simulink model "PubIfDecisionTOS_MDL"  (R2020b)
settings: configuration reference "DspaceConfig" (kept outside this file)
PostLoadFcn:
  | if any(exist('dsrtsu_mdlpostloadfcn', 'file') ~= 0), dsrtsu_mdlpostloadfcn('Execute', bdroot); end
InitFcn:
  | , if any(exist('dsmpb_private', 'file') ~= 0), dsmpb_private('dsmpb_mdlclblib', 'Init', bdroot); end,
undefined symbols (not defined in the file or in its folder): C_TOS_ACCEgoRAxletoFbumplength_m, C_TOS_ACCTargetFront_Flag, C_TOS_AEBJAPedObjDxThre_Val, C_TOS_AEBJAPedObjDyThre_Val, C_TOS_AEBJATargetSize_Val, C_TOS_AEBJAVehObjDxThre_Val, C_TOS_AEBJAVehObjDyThre_Val, C_TOS_AEBJuncPedTargetSize_Val, C_TOS_AEBLatObjDxThre_Val, C_TOS_AEBLatPedDyThre_Val, C_TOS_AEBLatTargetSize_Val, C_TOS_AEBLongTargetInEgoFront_Flag, C_TOS_axAbsGround_Parameter, C_TOS_CameraConfirmedFlag, C_TOS_CNsubjWidth, C_TOS_CurrentLaneCoreMinWidth_Val, C_TOS_CutInProb_Val_Zero, C_TOS_CutOutProb_Val_Zero, C_TOS_D2R_Val, C_TOS_DefaultValueObjectToCenterLine_dy, C_TOS_EgoCarWidth_Val, C_TOS_EgoDxRefPoint_m, C_TOS_EgoRAxletoFbumplength_m, C_TOS_HalfWidthVehicle_Con, C_TOS_HWA_CurrentLaneFlag, C_TOS_HWA_LeftLaneFlag, C_TOS_HWA_MovingDir_Vaild, C_TOS_HWA_MovState_Vaild, C_TOS_HWA_RightLaneFlag, C_TOS_LaneLineCourseErrorFront, C_TOS_LaneLineCourseErrorRear, C_TOS_MotorbikeDefaultWidth_m, C_TOS_NumberOfEffectiveTargets, C_TOS_Obj_Age_Val, C_TOS_Objdx_Constraint_Val, C_TOS_ObjectDefaultWidth_m, C_TOS_ObjInCurrentLane_Val, C_TOS_ObjInCurrentLaneValid, C_TOS_ObjInLeftLaneValid, C_TOS_ObjInRightLaneValid, C_TOS_ObjNotInCurrentLane_Val, C_TOS_ObjNotREElementType, C_TOS_ObjPredictDis_dy_ConstantVal_Zeros, C_TOS_ObjToCenterLine_ConstantVal_Zeros, C_TOS_OFMObjIDInvilad_Val, C_TOS_PIL_LatDisCons_Val_zero, C_TOS_PIL_ObjectCutInFlag_b, C_TOS_PIL_ObjectCutOutFlag_b, C_TOS_PIL_ObjLaneProb_al_Val, C_TOS_PP_ObjFusType_FC_Confirm_b, C_TOS_PP_ObjFusType_FC_FR_Confirm_b, C_TOS_PP_ObjFusType_FR_Confirm_b, C_TOS_RE_80BoolDefault_Val, C_TOS_RE_80Single181Default_Val, C_TOS_RE_80Single255Default_Val, C_TOS_RE_80Uint8Default_Val, C_TOS_RE_D2R, C_TOS_RE_D_180_Val, C_TOS_RE_InvalidObjectID_Val, C_TOS_RE_InvalidTargetChainDir_Val ... (+142)
libraries: simulink x1650, TOS_LIB x361, canfdmsglib x14
(part 17 of 69)

== system PubIfDecisionTOS_MDL/TOS_20201112/TOS_2012080320/PP1128/AAT-AdditionalAttributes/PP_ObjectToCenterLine_dy/PP_ObjectToCenterLine_vyc/PP_ObjectToCenterLine_vyc_Filt ==
  TOS_OFMObjValid_Flag : Inport
  Object_ID : Inport  Port=2  OutDataTypeStr=uint8
  Object_Age : Inport  Port=3
  PP_ObjectToCenterLine_vyc : Inport  Port=4
  ObjectToCenterLine_vyc : Subsystem
  Unit Delay : UnitDelay  InitialCondition=zeros(80,1)  SampleTime=-1  HasFrameUpgradeWarning=on
      settings: AttributesFormatString=initVal = zeros(80,1)
  Unit Delay1 : UnitDelay  InitialCondition=ones(80,1)*255  SampleTime=-1  HasFrameUpgradeWarning=on
      settings: AttributesFormatString=initVal = ones(80,1)*255
  PP_ObjectToCenterLine_vyc_Filt : Outport  OutDataTypeStr=single
  wires:
  TOS_OFMObjValid_Flag/1 -> ObjectToCenterLine_vyc/4(TOS_OFMObjValid_Flag)
  Object_Age/1 -> ObjectToCenterLine_vyc/6(Object_Age)
  PP_ObjectToCenterLine_vyc/1 -> ObjectToCenterLine_vyc/3(PP_ObjectToCenterLine_vyc)
  ObjectToCenterLine_vyc/2(PP_ObjectToCenterLine_vyc_Filt) -> PP_ObjectToCenterLine_vyc_Filt/1, Unit Delay1/1
  Unit Delay1/1 -> ObjectToCenterLine_vyc/2(PP_ObjectToCenterLine_vyc_Filt_K1)
  Object_ID/1 -> ObjectToCenterLine_vyc/5(Object_ID)
  ObjectToCenterLine_vyc/1(Obj_ID) -> Unit Delay/1
  Unit Delay/1 -> ObjectToCenterLine_vyc/1(ObjectID_Filt_K1)

== system PubIfDecisionTOS_MDL/TOS_20201112/TOS_2012080320/PP1128/AAT-AdditionalAttributes/PP_SignalProcessing/PP_SignalProcessing/CamareConfirmSignalProcessing ==
  note: PP_CamareConfirmSignalProcessing
      |
      | 是否摄像头确认信号（AEB）
      |
      | fun1:有摄像头、前雷达参与
  Object_FusType : Inport
  Data Type Conversion : DataTypeConversion  OutDataTypeStr=Enum: OFM_OBJ_FUSTYPE
  Enumerated Constant : simulink/Sources/Enumerated Constant  OutDataTypeStr=Enum: OFM_OBJ_FUSTYPE  Value=OFM_OBJ_FUSTYPE.FC_FR  SampleTime=inf
      settings: AttributesFormatString=OFM_OBJ_FUSTYPE.FC_FR = 3
  Enumerated Constant1 : simulink/Sources/Enumerated Constant  OutDataTypeStr=Enum: OFM_OBJ_FUSTYPE  Value=OFM_OBJ_FUSTYPE.FC_FR_CL  SampleTime=inf
      settings: AttributesFormatString=OFM_OBJ_FUSTYPE.FC_FR_CL=7
  Enumerated Constant10 : simulink/Sources/Enumerated Constant  OutDataTypeStr=Enum: OFM_OBJ_FUSTYPE  Value=OFM_OBJ_FUSTYPE.FC_FR_CR_BR  SampleTime=inf
      settings: AttributesFormatString=OFM_OBJ_FUSTYPE.FC_FR_CR_BR=43
  Enumerated Constant11 : simulink/Sources/Enumerated Constant  OutDataTypeStr=Enum: OFM_OBJ_FUSTYPE  Value=OFM_OBJ_FUSTYPE.FC_FR_CL_CR_BR  SampleTime=inf
      settings: AttributesFormatString=OFM_OBJ_FUSTYPE.FC_FR_CL_CR_BR=47
  Enumerated Constant12 : simulink/Sources/Enumerated Constant  OutDataTypeStr=Enum: OFM_OBJ_FUSTYPE  Value=OFM_OBJ_FUSTYPE.FC_FR_BL_BR  SampleTime=inf
      settings: AttributesFormatString=OFM_OBJ_FUSTYPE.FC_FR_BL_BR=51
  Enumerated Constant13 : simulink/Sources/Enumerated Constant  OutDataTypeStr=Enum: OFM_OBJ_FUSTYPE  Value=OFM_OBJ_FUSTYPE.FC_FR_CR_BL_BR  SampleTime=inf
      settings: AttributesFormatString=OFM_OBJ_FUSTYPE.FC_FR_CR_BL_BR=59
  Enumerated Constant14 : simulink/Sources/Enumerated Constant  OutDataTypeStr=Enum: OFM_OBJ_FUSTYPE  Value=OFM_OBJ_FUSTYPE.FC_FR_CL_BL_BR  SampleTime=inf
      settings: AttributesFormatString=OFM_OBJ_FUSTYPE.FC_FR_CL_BL_BR=55
  Enumerated Constant15 : simulink/Sources/Enumerated Constant  OutDataTypeStr=Enum: OFM_OBJ_FUSTYPE  Value=OFM_OBJ_FUSTYPE.FC_FR_CL_CR_BL_BR  SampleTime=inf
      settings: AttributesFormatString=OFM_OBJ_FUSTYPE.FC_FR_CL_CR_BL_BR=63
  Enumerated Constant2 : simulink/Sources/Enumerated Constant  OutDataTypeStr=Enum: OFM_OBJ_FUSTYPE  Value=OFM_OBJ_FUSTYPE.FC_FR_CR  SampleTime=inf
      settings: AttributesFormatString=OFM_OBJ_FUSTYPE.FC_FR_CR=11
  Enumerated Constant3 : simulink/Sources/Enumerated Constant  OutDataTypeStr=Enum: OFM_OBJ_FUSTYPE  Value=OFM_OBJ_FUSTYPE.FC_FR_CL_CR  SampleTime=inf
      settings: AttributesFormatString=OFM_OBJ_FUSTYPE.FC_FR_CL_CR=15
  Enumerated Constant4 : simulink/Sources/Enumerated Constant  OutDataTypeStr=Enum: OFM_OBJ_FUSTYPE  Value=OFM_OBJ_FUSTYPE.FC_FR_BL  SampleTime=inf
      settings: AttributesFormatString=OFM_OBJ_FUSTYPE.FC_FR_BL=19
  Enumerated Constant5 : simulink/Sources/Enumerated Constant  OutDataTypeStr=Enum: OFM_OBJ_FUSTYPE  Value=OFM_OBJ_FUSTYPE.FC_FR_CL_BL  SampleTime=inf
      settings: AttributesFormatString=OFM_OBJ_FUSTYPE.FC_FR_CL_BL=23
  Enumerated Constant6 : simulink/Sources/Enumerated Constant  OutDataTypeStr=Enum: OFM_OBJ_FUSTYPE  Value=OFM_OBJ_FUSTYPE.FC_FR_CR_BL  SampleTime=inf
      settings: AttributesFormatString=OFM_OBJ_FUSTYPE.FC_FR_CR_BL=27
  Enumerated Constant7 : simulink/Sources/Enumerated Constant  OutDataTypeStr=Enum: OFM_OBJ_FUSTYPE  Value=OFM_OBJ_FUSTYPE.FC_FR_CL_CR_BL  SampleTime=inf
      settings: AttributesFormatString=OFM_OBJ_FUSTYPE.FC_FR_CL_CR_BL=31
  Enumerated Constant8 : simulink/Sources/Enumerated Constant  OutDataTypeStr=Enum: OFM_OBJ_FUSTYPE  Value=OFM_OBJ_FUSTYPE.FC_FR_BR  SampleTime=inf
      settings: AttributesFormatString=OFM_OBJ_FUSTYPE.FC_FR_BR=35
  Enumerated Constant9 : simulink/Sources/Enumerated Constant  OutDataTypeStr=Enum: OFM_OBJ_FUSTYPE  Value=OFM_OBJ_FUSTYPE.FC_FR_CL_BR  SampleTime=inf
      settings: AttributesFormatString=OFM_OBJ_FUSTYPE.FC_FR_CL_BR=39
  Logical Operator{1..15} (15 alike) : Logic  Operator=OR  AllPortsSameDT=off  OutDataTypeStr=boolean
  Relational Operator{1..16} (16 alike) : RelationalOperator  Operator===  OutDataTypeStr=boolean  RndMeth=Nearest
  PP_CamareConfirmSignalProcessing : Outport
  wires:
  Enumerated Constant1/1 -> Relational Operator12/2
  Relational Operator12/1 -> Logical Operator8/2
  Enumerated Constant2/1 -> Relational Operator13/2
  Enumerated Constant3/1 -> Relational Operator15/2
  Relational Operator15/1 -> Logical Operator9/2
  Relational Operator14/1 -> Logical Operator8/1
  Logical Operator15/1 -> PP_CamareConfirmSignalProcessing/1
  Relational Operator13/1 -> Logical Operator9/1
  Logical Operator8/1 -> Logical Operator10/1
  Logical Operator9/1 -> Logical Operator10/2
  Enumerated Constant/1 -> Relational Operator14/2
  Object_FusType/1 -> Data Type Conversion/1
  Enumerated Constant4/1 -> Relational Operator3/2
  Enumerated Constant7/1 -> Relational Operator4/2
  Enumerated Constant6/1 -> Relational Operator2/2
  Enumerated Constant5/1 -> Relational Operator1/2
  Enumerated Constant9/1 -> Relational Operator5/2
  Enumerated Constant10/1 -> Relational Operator6/2
  Enumerated Constant11/1 -> Relational Operator8/2
  Enumerated Constant8/1 -> Relational Operator7/2
  Enumerated Constant12/1 -> Relational Operator11/2
  Enumerated Constant15/1 -> Relational Operator16/2
  Data Type Conversion/1 -> Relational Operator14/1, Relational Operator12/1, Relational Operator3/1, Relational Operator1/1, Relational Operator2/1, Relational Operator4/1, Relational Operator7/1, Relational Operator5/1, Relational Operator6/1, Relational Operator8/1, Relational Operator11/1, Relational Operator9/1, Relational Operator10/1, Relational Operator16/1, Relational Operator15/1, Relational Operator13/1
  Enumerated Constant13/1 -> Relational Operator10/2
  Enumerated Constant14/1 -> Relational Operator9/2
  Relational Operator3/1 -> Logical Operator1/1
  Relational Operator1/1 -> Logical Operator1/2
  Relational Operator2/1 -> Logical Operator2/1
  Relational Operator4/1 -> Logical Operator2/2
  Relational Operator9/1 -> Logical Operator4/2
  Relational Operator11/1 -> Logical Operator4/1
  Relational Operator8/1 -> Logical Operator3/2
  Relational Operator6/1 -> Logical Operator3/1
  Relational Operator7/1 -> Logical Operator5/1
  Relational Operator5/1 -> Logical Operator5/2
  Relational Operator10/1 -> Logical Operator6/1
  Relational Operator16/1 -> Logical Operator6/2
  Logical Operator2/1 -> Logical Operator12/2
  Logical Operator1/1 -> Logical Operator12/1
  Logical Operator5/1 -> Logical Operator13/1
  Logical Operator3/1 -> Logical Operator13/2
  Logical Operator6/1 -> Logical Operator7/2
  Logical Operator4/1 -> Logical Operator7/1
  Logical Operator10/1 -> Logical Operator11/1
  Logical Operator12/1 -> Logical Operator11/2
  Logical Operator13/1 -> Logical Operator14/1
  Logical Operator7/1 -> Logical Operator14/2
  Logical Operator11/1 -> Logical Operator15/1
  Logical Operator14/1 -> Logical Operator15/2

== system PubIfDecisionTOS_MDL/TOS_20201112/TOS_2012080320/PP1128/AAT-AdditionalAttributes/PP_SignalProcessing/PP_SignalProcessing/MovingState_SignalProcessing ==
  Object_MovingState : Inport
  MovingState_SignalProcessing_V2011120315 : Subsystem
  MovingState_SignalProcessing_V2011130316 : Subsystem
  PP_MovingStateSignalProcessing : Outport
  PP_MovingState_AEB_SignalProcessing : Outport  Port=2
  wires:
  MovingState_SignalProcessing_V2011130316/1(PP_MovingStateSignalProcessing) -> PP_MovingStateSignalProcessing/1
  Object_MovingState/1 -> MovingState_SignalProcessing_V2011120315/1(Object_MovingState), MovingState_SignalProcessing_V2011130316/1(Object_MovingState)
  MovingState_SignalProcessing_V2011120315/1(PP_MovingStateSignalProcessing) -> PP_MovingState_AEB_SignalProcessing/1

== system PubIfDecisionTOS_MDL/TOS_20201112/TOS_2012080320/PP1128/AAT-AdditionalAttributes/PP_SignalProcessing/PP_SignalProcessing/ObjFusTypeConfirm ==
  Object_FusType : Inport
  Data Type Conversion : DataTypeConversion  OutDataTypeStr=Enum: OFM_OBJ_FUSTYPE
  FC_FR_other : Subsystem
  FC_other : Subsystem
  FR_other : Subsystem
  ObjFusType : Subsystem  Commented=on
  ObjFusType_FC_FR_Confirm : Outport
  ObjFusType_FR_Confirm : Outport  Port=2
  ObjFusType_FC_Confirm : Outport  Port=3
  wires:
  Object_FusType/1 -> Data Type Conversion/1
  Data Type Conversion/1 -> FC_other/1(Object_FusType), FR_other/1(Object_FusType), FC_FR_other/1(Object_FusType)
  FC_FR_other/1(FC_FR_other) -> ObjFusType_FC_FR_Confirm/1
  FR_other/1(FR_Other) -> ObjFusType_FR_Confirm/1
  FC_other/1(FC_other) -> ObjFusType_FC_Confirm/1

== system PubIfDecisionTOS_MDL/TOS_20201112/TOS_2012080320/PP1128/AAT-AdditionalAttributes/PP_SignalProcessing/PP_SignalProcessing/ObjMovingDirSignalProcessing ==
  Object_MovingOrientation : Inport
  Compare To Constant : simulink/Logic and Bit Operations/Compare To Constant  relop===  const=OFM_OBJ_ORIENTATION_E.NORTH  OutDataTypeStr=boolean
      settings: AttributesFormatString=OFM_OBJ_ORIENTATION_E.NORTH = 9
  Compare To Constant3 : simulink/Logic and Bit Operations/Compare To Constant  relop===  const=OFM_OBJ_ORIENTATION_E.SOUTH  OutDataTypeStr=boolean
      settings: AttributesFormatString=OFM_OBJ_ORIENTATION_E.SOUTH = 5
  Compare To Constant4 : simulink/Logic and Bit Operations/Compare To Constant  relop===  const=OFM_OBJ_ORIENTATION_E.WEST  OutDataTypeStr=boolean
      settings: AttributesFormatString=OFM_OBJ_ORIENTATION_E.WEST = 7
  Compare To Constant5 : simulink/Logic and Bit Operations/Compare To Constant  relop===  const=OFM_OBJ_ORIENTATION_E.EAST  OutDataTypeStr=boolean
      settings: AttributesFormatString=OFM_OBJ_ORIENTATION_E.EAST = 3
  Data Type Conversion1 : DataTypeConversion  OutDataTypeStr=uint8
  Data Type Conversion2 : DataTypeConversion  OutDataTypeStr=Enum: OFM_OBJ_ORIENTATION_E
  Enumerated Constant : simulink/Sources/Enumerated Constant  OutDataTypeStr=Enum: ObjectMovingOrientation_E  Value=ObjectMovingOrientation_E.SameDir  SampleTime=inf
      settings: AttributesFormatString=ObjectMovingOrientation_E.SameDir = 1
  Enumerated Constant1 : simulink/Sources/Enumerated Constant  OutDataTypeStr=Enum: ObjectMovingOrientation_E  Value=ObjectMovingOrientation_E.OnComingDir  SampleTime=inf
      settings: AttributesFormatString=ObjectMovingOrientation_E.OnComingDir = 2
  Enumerated Constant2 : simulink/Sources/Enumerated Constant  OutDataTypeStr=Enum: ObjectMovingOrientation_E  Value=ObjectMovingOrientation_E.Crossing  SampleTime=inf
      settings: AttributesFormatString=ObjectMovingOrientation_E.Crossing = 3
  Enumerated Constant3 : simulink/Sources/Enumerated Constant  OutDataTypeStr=Enum: ObjectMovingOrientation_E  Value=ObjectMovingOrientation_E.UnknownDir  SampleTime=inf
      settings: AttributesFormatString=ObjectMovingOrientation_E.UnknownDir = 0
  Logical Operator6 : Logic  Operator=OR  AllPortsSameDT=off  OutDataTypeStr=boolean
  Switch : Switch  Criteria=u2 ~= 0
  Switch1 : Switch  Criteria=u2 ~= 0
  Switch2 : Switch  Criteria=u2 ~= 0
  PP_ObjMovingDirSignalProcessing : Outport
  wires:
  Switch/1 -> Data Type Conversion1/1
  Enumerated Constant3/1 -> Switch2/3
  Switch1/1 -> Switch/3
  Switch2/1 -> Switch1/3
  Enumerated Constant2/1 -> Switch2/1
  Enumerated Constant1/1 -> Switch1/1
  Logical Operator6/1 -> Switch2/2
  Compare To Constant3/1 -> Switch1/2
  Compare To Constant4/1 -> Logical Operator6/1
  Data Type Conversion2/1 -> Compare To Constant/1, Compare To Constant3/1, Compare To Constant5/1, Compare To Constant4/1
  Compare To Constant5/1 -> Logical Operator6/2
  Enumerated Constant/1 -> Switch/1
  Compare To Constant/1 -> Switch/2
  Object_MovingOrientation/1 -> Data Type Conversion2/1
  Data Type Conversion1/1 -> PP_ObjMovingDirSignalProcessing/1

== system PubIfDecisionTOS_MDL/TOS_20201112/TOS_2012080320/PP1128/AAT-AdditionalAttributes/PP_SignalProcessing/PP_SignalProcessing/ObjToEgoCarFrontbump ==
  note: 目标到自车前保之间距离
  Object_Dx : Inport
  Constant1 : Constant  Value=C_TOS_ACCEgoRAxletoFbumplength_m  OutDataTypeStr=single
      settings: AttributesFormatString=C_TOS_ACCEgoRAxletoFbumplength_m = 3.93 m
  Subtract : Sum  Inputs=+-
  PP_ObjToEgoCarFrontbump : Outport
  wires:
  Object_Dx/1 -> Subtract/1
  Subtract/1 -> PP_ObjToEgoCarFrontbump/1
  Constant1/1 -> Subtract/2

== system PubIfDecisionTOS_MDL/TOS_20201112/TOS_2012080320/PP1128/AAT-AdditionalAttributes/PP_SignalProcessing/PP_SignalProcessing/axAbsGround ==
  note: Fun：计算目标相对于大地的绝对加速度(ACC)
      |
      | fun1:目标绝对加速度 = 目标相对加速度（融合输出）+ 自车加速度
      | fun2: 当目标状态为STATIONARY、STOPPED时，输出目标绝对加速度为0
      |
      |
      | （目标相对加速度 = 目标加速度 - 自车加速度）
  Object_AX : Inport
  axvRefMs2 : Inport  Port=2
  Object_MovingState : Inport  Port=3
  Add : Sum
  Compare To Constant : simulink/Logic and Bit Operations/Compare To Constant  relop===  const=OFM_OBJ_MOVINGSTATE_E.STATIONARY  OutDataTypeStr=boolean
      settings: AttributesFormatString=OFM_OBJ_MOVINGSTATE_E.STATIONARY = 3
  Compare To Constant1 : simulink/Logic and Bit Operations/Compare To Constant  relop===  const=OFM_OBJ_MOVINGSTATE_E.STOPPED  OutDataTypeStr=boolean
      settings: AttributesFormatString=OFM_OBJ_MOVINGSTATE_E.STOPPED = 4
  Constant1 : Constant  Value=C_TOS_axAbsGround_Parameter  OutDataTypeStr=single
      settings: AttributesFormatString=C_TOS_axAbsGround_Parameter = 0
  Data Type Conversion : DataTypeConversion  OutDataTypeStr=Enum: OFM_OBJ_MOVINGSTATE_E
  Logical Operator : Logic  Operator=OR  AllPortsSameDT=off  OutDataTypeStr=boolean
  Switch1 : Switch  Criteria=u2 ~= 0
  PP_axAbsGround : Outport
  wires:
  Compare To Constant1/1 -> Logical Operator/2
  axvRefMs2/1 -> Add/2
  Data Type Conversion/1 -> Compare To Constant1/1, Compare To Constant/1
  Object_AX/1 -> Add/1
  Compare To Constant/1 -> Logical Operator/1
  Object_MovingState/1 -> Data Type Conversion/1
  Switch1/1 -> PP_axAbsGround/1
  Constant1/1 -> Switch1/1
  Add/1 -> Switch1/3
  Logical Operator/1 -> Switch1/2

== system PubIfDecisionTOS_MDL/TOS_20201112/TOS_2012080320/PP1128/AAT-AdditionalAttributes/RoadEdge/RE_2020_12_07/RoadEdge_V2 ==
  OFM_Signal : Inport  BusOutputAsStruct=on
  vxvRefMs : Inport  Port=2  OutDataTypeStr=single  PortDimensions=1  BusOutputAsStruct=on
  Bus Selector : BusSelector  OutputSignals=RE_EgoLeftTargetChainStartIndex
  Bus Selector1 : BusSelector  OutputSignals=RE_EgoRightTargetChainStartIndex
  Bus Selector2 : BusSelector  OutputSignals=RE_EgoLeftEdgeGroupChainStartIndex
  Bus Selector3 : BusSelector  OutputSignals=RE_EgoRightEdgeGroupChainStartIndex
  Bus Selector4 : BusSelector  OutputSignals=RE_EgoRightStationaryObjectsSortIndex
  Bus Selector5 : BusSelector  OutputSignals=RE_EgoLeftStationaryObjectsSortIndex
  RoadEdgeElementFinalJudge : Subsystem
  RoadEdgeElementType : Subsystem
  RoadEdgeGroupChain : Subsystem
  SelectStationaryObjects : Subsystem
  TargetChain : Subsystem
  Unit Delay1 : UnitDelay  SampleTime=-1  HasFrameUpgradeWarning=on
  Unit Delay2 : UnitDelay  SampleTime=-1  HasFrameUpgradeWarning=on
  RE_EdgeElementType : Outport
  RE_StationaryObjectFlag : Outport  Port=2
  RE_EgoLeftTargetChainStartIndex : Outport  Port=3
  RE_EgoRightTargetChainStartIndex : Outport  Port=4
  RE_EgoLeftEdgeGroupChainStartIndex : Outport  Port=5
  RE_EgoRightEdgeGroupChainStartIndex : Outport  Port=6
  RE_EgoLeftStationaryObjectsSortIndex : Outport  Port=7
  RE_EgoRightStationaryObjectsSortIndex : Outport  Port=8
  RE_EdgeElementID : Outport  Port=9
  wires:
  vxvRefMs/1 -> RoadEdgeGroupChain/6(vxvRefMs), RoadEdgeElementFinalJudge/5(vxvRefMs)
  SelectStationaryObjects/1(RE_StationaryObjectsSortIndex) -> Bus Selector5/1, Bus Selector4/1, TargetChain/1(RE_StillObjectsSortIndex)  "RE_StationaryObjectsSortIndex"
  TargetChain/1(RE_StillObjectSortIndex) -> RoadEdgeGroupChain/1(RE_StillObjectSortIndex)  "RE_StillObjectSortIndex"
  TargetChain/2(RE_EgoLeftTargetChainInfor) -> RoadEdgeGroupChain/2(RE_EgoLeftTargetChainInfor), Bus Selector/1  "RE_EgoLeftTargetChainInfor"
  TargetChain/3(RE_EgoRightTargetChainInfor) -> RoadEdgeGroupChain/3(RE_EgoRightTargetChainInfor), Bus Selector1/1  "RE_EgoRightTargetChainInfor"
  TargetChain/4(RE_TargetTheta) -> RoadEdgeGroupChain/4(RE_TargetTheta)  "RE_TargetTheta"
  RoadEdgeGroupChain/1(RE_EgoLeftEdgeGroupChainInfor) -> Bus Selector2/1, RoadEdgeElementFinalJudge/1(RE_EgoLeftEdgeGroupChainInfor)  "RE_EgoLeftEdgeGroupChainInfor"
  RoadEdgeElementType/1(RE_EdgeElementType) -> RE_EdgeElementType/1  "RE_EdgeElementType"
  RoadEdgeGroupChain/2(RE_EgoRightEdgeGroupChainInfor) -> Bus Selector3/1, RoadEdgeElementFinalJudge/2(RE_EgoRightEdgeGroupChainInfor)  "RE_EgoRightEdgeGroupChainInfor"
  RoadEdgeGroupChain/3(RE_Target_Theta) -> RoadEdgeElementFinalJudge/3(RE_Target_Theta)  "RE_Target_Theta"
  RoadEdgeGroupChain/4(REStillObjectSortIndex) -> RoadEdgeElementFinalJudge/4(REStillObjectSortIndex)  "REStillObjectSortIndex"
  RoadEdgeElementFinalJudge/1(RE_EgoLeft_EdgeElementType) -> RoadEdgeElementType/1(RE_EgoLeft_EdgeElementType)  "RE_EgoLeft_EdgeElementType"
  RoadEdgeElementFinalJudge/2(RE_EgoRight_EdgeElementType) -> RoadEdgeElementType/2(RE_EgoRight_EdgeElementType)  "RE_EgoRight_EdgeElementType"
  SelectStationaryObjects/2(RE_StationaryObjectFlag) -> RE_StationaryObjectFlag/1
  Bus Selector/1 -> RE_EgoLeftTargetChainStartIndex/1  "<RE_EgoLeftTargetChainStartIndex>"
  Bus Selector1/1 -> RE_EgoRightTargetChainStartIndex/1  "<RE_EgoRightTargetChainStartIndex>"
  Bus Selector3/1 -> RE_EgoRightEdgeGroupChainStartIndex/1  "<RE_EgoRightEdgeGroupChainStartIndex>"
  Bus Selector2/1 -> RE_EgoLeftEdgeGroupChainStartIndex/1  "<RE_EgoLeftEdgeGroupChainStartIndex>"
  Bus Selector4/1 -> RE_EgoRightStationaryObjectsSortIndex/1  "<RE_EgoRightStationaryObjectsSortIndex>"
  Bus Selector5/1 -> RE_EgoLeftStationaryObjectsSortIndex/1  "<RE_EgoLeftStationaryObjectsSortIndex>"
  RoadEdgeElementType/2(RE_EdgeElementID) -> [RE_EdgeElementID], RE_EdgeElementID/1  "RE_EdgeElementID"
  RoadEdgeElementFinalJudge/3(RE_EgoLeft_EdgeElementID) -> RoadEdgeElementType/3(RE_EgoLeft_EdgeElementID)  "RE_EgoLeft_EdgeElementID"
  RoadEdgeElementFinalJudge/4(RE_EgoRight_EdgeElementID) -> RoadEdgeElementType/4(RE_EgoRight_EdgeElementID)  "RE_EgoRight_EdgeElementID"
  OFM_Signal/1 -> RoadEdgeGroupChain/5(OFM_Signal), RoadEdgeElementType/5(OFM_Signal), RoadEdgeElementFinalJudge/7(OFM_Signal), TargetChain/2(OFM_Signal), SelectStationaryObjects/1(OFM_Signal)
  [RE_EdgeElementID] -> Unit Delay2/1
  [RE_EdgeElementID] -> Unit Delay1/1
  Unit Delay2/1 -> TargetChain/3(RE_EdgeElementID_K1)
  Unit Delay1/1 -> RoadEdgeElementFinalJudge/6(RE_EdgeElementID_K1)

== system PubIfDecisionTOS_MDL/TOS_20201112/TOS_2012080320/PP1128/AAT-AdditionalAttributes/TAP_TargetPreprocessing/TargetValidConfirm/TOS_OFMObjValidConfirm ==
  Object_ID : Inport  Partition=on  PartitionDimension=1  PartitionWidth=1  PartitionOffset=0
  Object_ObstacleProb : Inport  Port=2  Partition=on  PartitionDimension=1  PartitionWidth=1  PartitionOffset=0
  Object_ExistProb : Inport  Port=3  Partition=on  PartitionDimension=1  PartitionWidth=1  PartitionOffset=0
  Object_MovingState : Inport  Port=4  Partition=on  PartitionDimension=1  PartitionWidth=1  PartitionOffset=0
  Object_Type : Inport  Port=5  Partition=on  PartitionDimension=1  PartitionWidth=1  PartitionOffset=0
  Object_Age : Inport  Port=6  Partition=on  PartitionDimension=1  PartitionWidth=1  PartitionOffset=0
  Compare To Constant : simulink/Logic and Bit Operations/Compare To Constant  relop=>=  const=P_TOS_TAP_ObstacleProbThre_Valu  OutDataTypeStr=boolean
      settings: AttributesFormatString=P_TOS_TAP_ObstacleProbThre_Valu = 0.43
  Compare To Constant1 : simulink/Logic and Bit Operations/Compare To Constant  relop=>=  const=P_TOS_TAP_ExistProbThre_Valu  OutDataTypeStr=boolean
      settings: AttributesFormatString=P_TOS_TAP_ExistProbThre_Valu = 0.5
  Compare To Constant3 : simulink/Logic and Bit Operations/Compare To Constant  relop=~=  const=C_TOS_OFMObjIDInvilad_Val  OutDataTypeStr=boolean
      settings: AttributesFormatString=C_TOS_OFMObjIDInvilad_Val = 0
  For Each : ForEach  DisableCoverage=on
  Logical Operator1 : Logic  Inputs=3  AllPortsSameDT=off  OutDataTypeStr=boolean
  Terminator : Terminator
  Terminator1 : Terminator
  Terminator2 : Terminator
  TOS_OFMObjValid_Flag : Outport  ConcatenationDimension=1
  wires:
  Object_Age/1 -> Terminator2/1
  Object_Type/1 -> Terminator1/1
  Object_MovingState/1 -> Terminator/1
  Compare To Constant3/1 -> Logical Operator1/1
  Object_ID/1 -> Compare To Constant3/1
  Compare To Constant1/1 -> Logical Operator1/3
  Object_ExistProb/1 -> Compare To Constant1/1
  Compare To Constant/1 -> Logical Operator1/2
  Object_ObstacleProb/1 -> Compare To Constant/1
  Logical Operator1/1 -> TOS_OFMObjValid_Flag/1

== system PubIfDecisionTOS_MDL/TOS_20201112/TOS_2012080320/PP1128/ISV_InputSignalVerification/LM_SignalVerif/LM_LL_Bus/LM_LL_Line01 ==
  LM_Line01 : Inport
  Bus Creator2 : BusCreator  Inputs=8  OutDataTypeStr=Bus: TOS_LM_Line_bus  NonVirtualBus=on
      settings: InheritFromInputs=off
  Bus Selector2 : BusSelector  OutputSignals=pC0,pC1,pC2,pC3,dDisStart,dDisEnd,dQuality,fCamValid
  Signal Copy{1..7,24} (8 alike) : SignalConversion  OverrideOpt=off
  LM_LL_Line01 : Outport
  wires:
  Signal Copy1/1 -> Bus Creator2/2  "pC1"
  Bus Selector2/4 -> Signal Copy2/1  "<pC3>"
  Bus Creator2/1 -> LM_LL_Line01/1
  Signal Copy3/1 -> Bus Creator2/3  "pC2"
  Signal Copy6/1 -> Bus Creator2/5  "dDisStart"
  Signal Copy24/1 -> Bus Creator2/1  "pC0"
  Bus Selector2/1 -> Signal Copy24/1  "<pC0>"
  LM_Line01/1 -> Bus Selector2/1
  Bus Selector2/3 -> Signal Copy3/1  "<pC2>"
  Signal Copy4/1 -> Bus Creator2/6  "dDisEnd"
  Bus Selector2/5 -> Signal Copy6/1  "<dDisStart>"
  Bus Selector2/6 -> Signal Copy4/1  "<dDisEnd>"
  Bus Selector2/7 -> Signal Copy7/1  "<dQuality>"
  Bus Selector2/2 -> Signal Copy1/1  "<pC1>"
  Bus Selector2/8 -> Signal Copy5/1  "<fCamValid>"
  Signal Copy7/1 -> Bus Creator2/7  "dQuality"
  Signal Copy5/1 -> Bus Creator2/8  "fCamValid"
  Signal Copy2/1 -> Bus Creator2/4  "pC3"

== system PubIfDecisionTOS_MDL/TOS_20201112/TOS_2012080320/PP1128/ISV_InputSignalVerification/LM_SignalVerif/LM_LL_Bus/LM_LL_Line02 ==
  LM_Line02 : Inport
  Bus Creator2 : BusCreator  Inputs=8  OutDataTypeStr=Bus: TOS_LM_Line_bus  NonVirtualBus=on
      settings: InheritFromInputs=off
  Bus Selector2 : BusSelector  OutputSignals=pC0,pC1,pC2,pC3,dDisStart,dDisEnd,dQuality,fCamValid
  Signal Copy{1..7,24} (8 alike) : SignalConversion  OverrideOpt=off
  LM_LL_Line02 : Outport
  wires:
  Signal Copy2/1 -> Bus Creator2/4  "pC3"
  Signal Copy5/1 -> Bus Creator2/8  "fCamValid"
  Signal Copy7/1 -> Bus Creator2/7  "dQuality"
  Bus Selector2/8 -> Signal Copy5/1  "<fCamValid>"
  Bus Selector2/2 -> Signal Copy1/1  "<pC1>"
  Bus Selector2/7 -> Signal Copy7/1  "<dQuality>"
  Bus Selector2/6 -> Signal Copy4/1  "<dDisEnd>"
  Bus Selector2/5 -> Signal Copy6/1  "<dDisStart>"
  Signal Copy4/1 -> Bus Creator2/6  "dDisEnd"
  Bus Selector2/3 -> Signal Copy3/1  "<pC2>"
  LM_Line02/1 -> Bus Selector2/1
  Bus Selector2/1 -> Signal Copy24/1  "<pC0>"
  Signal Copy24/1 -> Bus Creator2/1  "pC0"
  Signal Copy6/1 -> Bus Creator2/5  "dDisStart"
  Signal Copy3/1 -> Bus Creator2/3  "pC2"
  Bus Creator2/1 -> LM_LL_Line02/1
  Bus Selector2/4 -> Signal Copy2/1  "<pC3>"
  Signal Copy1/1 -> Bus Creator2/2  "pC1"

== system PubIfDecisionTOS_MDL/TOS_20201112/TOS_2012080320/PP1128/ISV_InputSignalVerification/LM_SignalVerif/LM_LL_Bus/LM_LL_Line03 ==
  LM_Line03 : Inport
  Bus Creator2 : BusCreator  Inputs=8  OutDataTypeStr=Bus: TOS_LM_Line_bus  NonVirtualBus=on
      settings: InheritFromInputs=off
  Bus Selector2 : BusSelector  OutputSignals=pC0,pC1,pC2,pC3,dDisStart,dDisEnd,dQuality,fCamValid
  Signal Copy{1..7,24} (8 alike) : SignalConversion  OverrideOpt=off
  LM_LL_Line03 : Outport
  wires:
  Signal Copy1/1 -> Bus Creator2/2  "pC1"
  Bus Selector2/4 -> Signal Copy2/1  "<pC3>"
  Bus Creator2/1 -> LM_LL_Line03/1
  Signal Copy3/1 -> Bus Creator2/3  "pC2"
  Signal Copy6/1 -> Bus Creator2/5  "dDisStart"
  Signal Copy24/1 -> Bus Creator2/1  "pC0"
  Bus Selector2/1 -> Signal Copy24/1  "<pC0>"
  LM_Line03/1 -> Bus Selector2/1
  Bus Selector2/3 -> Signal Copy3/1  "<pC2>"
  Signal Copy4/1 -> Bus Creator2/6  "dDisEnd"
  Bus Selector2/5 -> Signal Copy6/1  "<dDisStart>"
  Bus Selector2/6 -> Signal Copy4/1  "<dDisEnd>"
  Bus Selector2/7 -> Signal Copy7/1  "<dQuality>"
  Bus Selector2/2 -> Signal Copy1/1  "<pC1>"
  Bus Selector2/8 -> Signal Copy5/1  "<fCamValid>"
  Signal Copy7/1 -> Bus Creator2/7  "dQuality"
  Signal Copy5/1 -> Bus Creator2/8  "fCamValid"
  Signal Copy2/1 -> Bus Creator2/4  "pC3"

== system PubIfDecisionTOS_MDL/TOS_20201112/TOS_2012080320/PP1128/ISV_InputSignalVerification/LM_SignalVerif/LM_LL_Bus/LM_LL_Line04 ==
  LM_Line04 : Inport
  Bus Creator2 : BusCreator  Inputs=8  OutDataTypeStr=Bus: TOS_LM_Line_bus  NonVirtualBus=on
      settings: InheritFromInputs=off
  Bus Selector2 : BusSelector  OutputSignals=pC0,pC1,pC2,pC3,dDisStart,dDisEnd,dQuality,fCamValid
  Signal Copy{1..7,24} (8 alike) : SignalConversion  OverrideOpt=off
  LM_LL_Line04 : Outport
  wires:
  Signal Copy2/1 -> Bus Creator2/4  "pC3"
  Signal Copy5/1 -> Bus Creator2/8  "fCamValid"
  Signal Copy7/1 -> Bus Creator2/7  "dQuality"
  Bus Selector2/8 -> Signal Copy5/1  "<fCamValid>"
  Bus Selector2/2 -> Signal Copy1/1  "<pC1>"
  Bus Selector2/7 -> Signal Copy7/1  "<dQuality>"
  Bus Selector2/6 -> Signal Copy4/1  "<dDisEnd>"
  Bus Selector2/5 -> Signal Copy6/1  "<dDisStart>"
  Signal Copy4/1 -> Bus Creator2/6  "dDisEnd"
  Bus Selector2/3 -> Signal Copy3/1  "<pC2>"
  LM_Line04/1 -> Bus Selector2/1
  Bus Selector2/1 -> Signal Copy24/1  "<pC0>"
  Signal Copy24/1 -> Bus Creator2/1  "pC0"
  Signal Copy6/1 -> Bus Creator2/5  "dDisStart"
  Signal Copy3/1 -> Bus Creator2/3  "pC2"
  Bus Creator2/1 -> LM_LL_Line04/1
  Bus Selector2/4 -> Signal Copy2/1  "<pC3>"
  Signal Copy1/1 -> Bus Creator2/2  "pC1"

== system PubIfDecisionTOS_MDL/TOS_20201112/TOS_2012080320/PP1128/ISV_InputSignalVerification/LM_SignalVerif/LM_LL_Bus/LM_LL_Line05 ==
  LM_Line05 : Inport
  Bus Creator2 : BusCreator  Inputs=8  OutDataTypeStr=Bus: TOS_LM_Line_bus  NonVirtualBus=on
      settings: InheritFromInputs=off
  Bus Selector2 : BusSelector  OutputSignals=pC0,pC1,pC2,pC3,dDisStart,dDisEnd,dQuality,fCamValid
  Signal Copy{1..7,24} (8 alike) : SignalConversion  OverrideOpt=off
  LM_LL_Line05 : Outport
  wires:
  Signal Copy1/1 -> Bus Creator2/2  "pC1"
  Bus Selector2/4 -> Signal Copy2/1  "<pC3>"
  Bus Creator2/1 -> LM_LL_Line05/1
  Signal Copy3/1 -> Bus Creator2/3  "pC2"
  Signal Copy6/1 -> Bus Creator2/5  "dDisStart"
  Signal Copy24/1 -> Bus Creator2/1  "pC0"
  Bus Selector2/1 -> Signal Copy24/1  "<pC0>"
  LM_Line05/1 -> Bus Selector2/1
  Bus Selector2/3 -> Signal Copy3/1  "<pC2>"
  Signal Copy4/1 -> Bus Creator2/6  "dDisEnd"
  Bus Selector2/5 -> Signal Copy6/1  "<dDisStart>"
  Bus Selector2/6 -> Signal Copy4/1  "<dDisEnd>"
  Bus Selector2/7 -> Signal Copy7/1  "<dQuality>"
  Bus Selector2/2 -> Signal Copy1/1  "<pC1>"
  Bus Selector2/8 -> Signal Copy5/1  "<fCamValid>"
  Signal Copy7/1 -> Bus Creator2/7  "dQuality"
  Signal Copy5/1 -> Bus Creator2/8  "fCamValid"
  Signal Copy2/1 -> Bus Creator2/4  "pC3"

== system PubIfDecisionTOS_MDL/TOS_20201112/TOS_2012080320/PP1128/ISV_InputSignalVerification/LM_SignalVerif/LM_LL_Bus/LM_LL_Line06 ==
  LM_Line06 : Inport
  Bus Creator2 : BusCreator  Inputs=8  OutDataTypeStr=Bus: TOS_LM_Line_bus  NonVirtualBus=on
      settings: InheritFromInputs=off
  Bus Selector2 : BusSelector  OutputSignals=pC0,pC1,pC2,pC3,dDisStart,dDisEnd,dQuality,fCamValid
  Signal Copy{1..7,24} (8 alike) : SignalConversion  OverrideOpt=off
  LM_LL_Line06 : Outport
  wires:
  Signal Copy2/1 -> Bus Creator2/4  "pC3"
  Signal Copy5/1 -> Bus Creator2/8  "fCamValid"
  Signal Copy7/1 -> Bus Creator2/7  "dQuality"
  Bus Selector2/8 -> Signal Copy5/1  "<fCamValid>"
  Bus Selector2/2 -> Signal Copy1/1  "<pC1>"
  Bus Selector2/7 -> Signal Copy7/1  "<dQuality>"
  Bus Selector2/6 -> Signal Copy4/1  "<dDisEnd>"
  Bus Selector2/5 -> Signal Copy6/1  "<dDisStart>"
  Signal Copy4/1 -> Bus Creator2/6  "dDisEnd"
  Bus Selector2/3 -> Signal Copy3/1  "<pC2>"
  LM_Line06/1 -> Bus Selector2/1
  Bus Selector2/1 -> Signal Copy24/1  "<pC0>"
  Signal Copy24/1 -> Bus Creator2/1  "pC0"
  Signal Copy6/1 -> Bus Creator2/5  "dDisStart"
  Signal Copy3/1 -> Bus Creator2/3  "pC2"
  Bus Creator2/1 -> LM_LL_Line06/1
  Bus Selector2/4 -> Signal Copy2/1  "<pC3>"
  Signal Copy1/1 -> Bus Creator2/2  "pC1"

== system PubIfDecisionTOS_MDL/TOS_20201112/TOS_2012080320/PP1128/ISV_InputSignalVerification/LM_SignalVerif/LM_LL_Bus/LM_LL_Line07 ==
  LM_Line07 : Inport
  Bus Creator2 : BusCreator  Inputs=8  OutDataTypeStr=Bus: TOS_LM_Line_bus  NonVirtualBus=on
      settings: InheritFromInputs=off
  Bus Selector2 : BusSelector  OutputSignals=pC0,pC1,pC2,pC3,dDisStart,dDisEnd,dQuality,fCamValid
  Signal Copy{1..7,24} (8 alike) : SignalConversion  OverrideOpt=off
  LM_LL_Line07 : Outport
  wires:
  Signal Copy1/1 -> Bus Creator2/2  "pC1"
  Bus Selector2/4 -> Signal Copy2/1  "<pC3>"
  Bus Creator2/1 -> LM_LL_Line07/1
  Signal Copy3/1 -> Bus Creator2/3  "pC2"
  Signal Copy6/1 -> Bus Creator2/5  "dDisStart"
  Signal Copy24/1 -> Bus Creator2/1  "pC0"
  Bus Selector2/1 -> Signal Copy24/1  "<pC0>"
  LM_Line07/1 -> Bus Selector2/1
  Bus Selector2/3 -> Signal Copy3/1  "<pC2>"
  Signal Copy4/1 -> Bus Creator2/6  "dDisEnd"
  Bus Selector2/5 -> Signal Copy6/1  "<dDisStart>"
  Bus Selector2/6 -> Signal Copy4/1  "<dDisEnd>"
  Bus Selector2/7 -> Signal Copy7/1  "<dQuality>"
  Bus Selector2/2 -> Signal Copy1/1  "<pC1>"
  Bus Selector2/8 -> Signal Copy5/1  "<fCamValid>"
  Signal Copy7/1 -> Bus Creator2/7  "dQuality"
  Signal Copy5/1 -> Bus Creator2/8  "fCamValid"
  Signal Copy2/1 -> Bus Creator2/4  "pC3"

== system PubIfDecisionTOS_MDL/TOS_20201112/TOS_2012080320/PP1128/ISV_InputSignalVerification/LM_SignalVerif/LM_LL_Bus/LM_LL_Line08 ==
  LM_Line08 : Inport
  Bus Creator2 : BusCreator  Inputs=8  OutDataTypeStr=Bus: TOS_LM_Line_bus  NonVirtualBus=on
      settings: InheritFromInputs=off
  Bus Selector2 : BusSelector  OutputSignals=pC0,pC1,pC2,pC3,dDisStart,dDisEnd,dQuality,fCamValid
  Signal Copy{1..7,24} (8 alike) : SignalConversion  OverrideOpt=off
  LM_LL_Line08 : Outport
  wires:
  Signal Copy2/1 -> Bus Creator2/4  "pC3"
  Signal Copy5/1 -> Bus Creator2/8  "fCamValid"
  Signal Copy7/1 -> Bus Creator2/7  "dQuality"
  Bus Selector2/8 -> Signal Copy5/1  "<fCamValid>"
  Bus Selector2/2 -> Signal Copy1/1  "<pC1>"
  Bus Selector2/7 -> Signal Copy7/1  "<dQuality>"
  Bus Selector2/6 -> Signal Copy4/1  "<dDisEnd>"
  Bus Selector2/5 -> Signal Copy6/1  "<dDisStart>"
  Signal Copy4/1 -> Bus Creator2/6  "dDisEnd"
  Bus Selector2/3 -> Signal Copy3/1  "<pC2>"
  LM_Line08/1 -> Bus Selector2/1
  Bus Selector2/1 -> Signal Copy24/1  "<pC0>"
  Signal Copy24/1 -> Bus Creator2/1  "pC0"
  Signal Copy6/1 -> Bus Creator2/5  "dDisStart"
  Signal Copy3/1 -> Bus Creator2/3  "pC2"
  Bus Creator2/1 -> LM_LL_Line08/1
  Bus Selector2/4 -> Signal Copy2/1  "<pC3>"
  Signal Copy1/1 -> Bus Creator2/2  "pC1"

== system PubIfDecisionTOS_MDL/TOS_20201112/TOS_2012080320/PP1128/ISV_InputSignalVerification/LM_SignalVerif/LM_LR_Bus/LM_LR_Line01 ==
  LM_Line01 : Inport
  Bus Creator2 : BusCreator  Inputs=8  OutDataTypeStr=Bus: TOS_LM_Line_bus  NonVirtualBus=on
      settings: InheritFromInputs=off
  Bus Selector2 : BusSelector  OutputSignals=pC0,pC1,pC2,pC3,dDisStart,dDisEnd,dQuality,fCamValid
  Signal Copy{1..7,24} (8 alike) : SignalConversion  OverrideOpt=off
  LM_LR_Line01 : Outport
  wires:
  Signal Copy2/1 -> Bus Creator2/4  "pC3"
  Signal Copy5/1 -> Bus Creator2/8  "fCamValid"
  Signal Copy7/1 -> Bus Creator2/7  "dQuality"
  Bus Selector2/8 -> Signal Copy5/1  "<fCamValid>"
  Bus Selector2/2 -> Signal Copy1/1  "<pC1>"
  Bus Selector2/7 -> Signal Copy7/1  "<dQuality>"
  Bus Selector2/6 -> Signal Copy4/1  "<dDisEnd>"
  Bus Selector2/5 -> Signal Copy6/1  "<dDisStart>"
  Signal Copy4/1 -> Bus Creator2/6  "dDisEnd"
  Bus Selector2/3 -> Signal Copy3/1  "<pC2>"
  LM_Line01/1 -> Bus Selector2/1
  Bus Selector2/1 -> Signal Copy24/1  "<pC0>"
  Signal Copy24/1 -> Bus Creator2/1  "pC0"
  Signal Copy6/1 -> Bus Creator2/5  "dDisStart"
  Signal Copy3/1 -> Bus Creator2/3  "pC2"
  Bus Creator2/1 -> LM_LR_Line01/1
  Bus Selector2/4 -> Signal Copy2/1  "<pC3>"
  Signal Copy1/1 -> Bus Creator2/2  "pC1"

== system PubIfDecisionTOS_MDL/TOS_20201112/TOS_2012080320/PP1128/ISV_InputSignalVerification/LM_SignalVerif/LM_LR_Bus/LM_LR_Line02 ==
  LM_Line02 : Inport
  Bus Creator2 : BusCreator  Inputs=8  OutDataTypeStr=Bus: TOS_LM_Line_bus  NonVirtualBus=on
      settings: InheritFromInputs=off
  Bus Selector2 : BusSelector  OutputSignals=pC0,pC1,pC2,pC3,dDisStart,dDisEnd,dQuality,fCamValid
  Signal Copy{1..7,24} (8 alike) : SignalConversion  OverrideOpt=off
  LM_LR_Line02 : Outport
  wires:
  Signal Copy1/1 -> Bus Creator2/2  "pC1"
  Bus Selector2/4 -> Signal Copy2/1  "<pC3>"
  Bus Creator2/1 -> LM_LR_Line02/1
  Signal Copy3/1 -> Bus Creator2/3  "pC2"
  Signal Copy6/1 -> Bus Creator2/5  "dDisStart"
  Signal Copy24/1 -> Bus Creator2/1  "pC0"
  Bus Selector2/1 -> Signal Copy24/1  "<pC0>"
  LM_Line02/1 -> Bus Selector2/1
  Bus Selector2/3 -> Signal Copy3/1  "<pC2>"
  Signal Copy4/1 -> Bus Creator2/6  "dDisEnd"
  Bus Selector2/5 -> Signal Copy6/1  "<dDisStart>"
  Bus Selector2/6 -> Signal Copy4/1  "<dDisEnd>"
  Bus Selector2/7 -> Signal Copy7/1  "<dQuality>"
  Bus Selector2/2 -> Signal Copy1/1  "<pC1>"
  Bus Selector2/8 -> Signal Copy5/1  "<fCamValid>"
  Signal Copy7/1 -> Bus Creator2/7  "dQuality"
  Signal Copy5/1 -> Bus Creator2/8  "fCamValid"
  Signal Copy2/1 -> Bus Creator2/4  "pC3"

== system PubIfDecisionTOS_MDL/TOS_20201112/TOS_2012080320/PP1128/ISV_InputSignalVerification/LM_SignalVerif/LM_LR_Bus/LM_LR_Line03 ==
  LM_Line03 : Inport
  Bus Creator2 : BusCreator  Inputs=8  OutDataTypeStr=Bus: TOS_LM_Line_bus  NonVirtualBus=on
      settings: InheritFromInputs=off
  Bus Selector2 : BusSelector  OutputSignals=pC0,pC1,pC2,pC3,dDisStart,dDisEnd,dQuality,fCamValid
  Signal Copy{1..7,24} (8 alike) : SignalConversion  OverrideOpt=off
  LM_LR_Line03 : Outport
  wires:
  Signal Copy2/1 -> Bus Creator2/4  "pC3"
  Signal Copy5/1 -> Bus Creator2/8  "fCamValid"
  Signal Copy7/1 -> Bus Creator2/7  "dQuality"
  Bus Selector2/8 -> Signal Copy5/1  "<fCamValid>"
  Bus Selector2/2 -> Signal Copy1/1  "<pC1>"
  Bus Selector2/7 -> Signal Copy7/1  "<dQuality>"
  Bus Selector2/6 -> Signal Copy4/1  "<dDisEnd>"
  Bus Selector2/5 -> Signal Copy6/1  "<dDisStart>"
  Signal Copy4/1 -> Bus Creator2/6  "dDisEnd"
  Bus Selector2/3 -> Signal Copy3/1  "<pC2>"
  LM_Line03/1 -> Bus Selector2/1
  Bus Selector2/1 -> Signal Copy24/1  "<pC0>"
  Signal Copy24/1 -> Bus Creator2/1  "pC0"
  Signal Copy6/1 -> Bus Creator2/5  "dDisStart"
  Signal Copy3/1 -> Bus Creator2/3  "pC2"
  Bus Creator2/1 -> LM_LR_Line03/1
  Bus Selector2/4 -> Signal Copy2/1  "<pC3>"
  Signal Copy1/1 -> Bus Creator2/2  "pC1"

== system PubIfDecisionTOS_MDL/TOS_20201112/TOS_2012080320/PP1128/ISV_InputSignalVerification/LM_SignalVerif/LM_LR_Bus/LM_LR_Line04 ==
  LM_Line04 : Inport
  Bus Creator2 : BusCreator  Inputs=8  OutDataTypeStr=Bus: TOS_LM_Line_bus  NonVirtualBus=on
      settings: InheritFromInputs=off
  Bus Selector2 : BusSelector  OutputSignals=pC0,pC1,pC2,pC3,dDisStart,dDisEnd,dQuality,fCamValid
  Signal Copy{1..7,24} (8 alike) : SignalConversion  OverrideOpt=off
  LM_LR_Line04 : Outport
  wires:
  Signal Copy1/1 -> Bus Creator2/2  "pC1"
  Bus Selector2/4 -> Signal Copy2/1  "<pC3>"
  Bus Creator2/1 -> LM_LR_Line04/1
  Signal Copy3/1 -> Bus Creator2/3  "pC2"
  Signal Copy6/1 -> Bus Creator2/5  "dDisStart"
  Signal Copy24/1 -> Bus Creator2/1  "pC0"
  Bus Selector2/1 -> Signal Copy24/1  "<pC0>"
  LM_Line04/1 -> Bus Selector2/1
  Bus Selector2/3 -> Signal Copy3/1  "<pC2>"
  Signal Copy4/1 -> Bus Creator2/6  "dDisEnd"
  Bus Selector2/5 -> Signal Copy6/1  "<dDisStart>"
  Bus Selector2/6 -> Signal Copy4/1  "<dDisEnd>"
  Bus Selector2/7 -> Signal Copy7/1  "<dQuality>"
  Bus Selector2/2 -> Signal Copy1/1  "<pC1>"
  Bus Selector2/8 -> Signal Copy5/1  "<fCamValid>"
  Signal Copy7/1 -> Bus Creator2/7  "dQuality"
  Signal Copy5/1 -> Bus Creator2/8  "fCamValid"
  Signal Copy2/1 -> Bus Creator2/4  "pC3"

== system PubIfDecisionTOS_MDL/TOS_20201112/TOS_2012080320/PP1128/ISV_InputSignalVerification/LM_SignalVerif/LM_LR_Bus/LM_LR_Line05 ==
  LM_Line05 : Inport
  Bus Creator2 : BusCreator  Inputs=8  OutDataTypeStr=Bus: TOS_LM_Line_bus  NonVirtualBus=on
      settings: InheritFromInputs=off
  Bus Selector2 : BusSelector  OutputSignals=pC0,pC1,pC2,pC3,dDisStart,dDisEnd,dQuality,fCamValid
  Signal Copy{1..7,24} (8 alike) : SignalConversion  OverrideOpt=off
  LM_LR_Line05 : Outport
  wires:
  Signal Copy2/1 -> Bus Creator2/4  "pC3"
  Signal Copy5/1 -> Bus Creator2/8  "fCamValid"
  Signal Copy7/1 -> Bus Creator2/7  "dQuality"
  Bus Selector2/8 -> Signal Copy5/1  "<fCamValid>"
  Bus Selector2/2 -> Signal Copy1/1  "<pC1>"
  Bus Selector2/7 -> Signal Copy7/1  "<dQuality>"
  Bus Selector2/6 -> Signal Copy4/1  "<dDisEnd>"
  Bus Selector2/5 -> Signal Copy6/1  "<dDisStart>"
  Signal Copy4/1 -> Bus Creator2/6  "dDisEnd"
  Bus Selector2/3 -> Signal Copy3/1  "<pC2>"
  LM_Line05/1 -> Bus Selector2/1
  Bus Selector2/1 -> Signal Copy24/1  "<pC0>"
  Signal Copy24/1 -> Bus Creator2/1  "pC0"
  Signal Copy6/1 -> Bus Creator2/5  "dDisStart"
  Signal Copy3/1 -> Bus Creator2/3  "pC2"
  Bus Creator2/1 -> LM_LR_Line05/1
  Bus Selector2/4 -> Signal Copy2/1  "<pC3>"
  Signal Copy1/1 -> Bus Creator2/2  "pC1"

== system PubIfDecisionTOS_MDL/TOS_20201112/TOS_2012080320/PP1128/ISV_InputSignalVerification/LM_SignalVerif/LM_LR_Bus/LM_LR_Line06 ==
  LM_Line06 : Inport
  Bus Creator2 : BusCreator  Inputs=8  OutDataTypeStr=Bus: TOS_LM_Line_bus  NonVirtualBus=on
      settings: InheritFromInputs=off
  Bus Selector2 : BusSelector  OutputSignals=pC0,pC1,pC2,pC3,dDisStart,dDisEnd,dQuality,fCamValid
  Signal Copy{1..7,24} (8 alike) : SignalConversion  OverrideOpt=off
  LM_LR_Line06 : Outport
  wires:
  Signal Copy1/1 -> Bus Creator2/2  "pC1"
  Bus Selector2/4 -> Signal Copy2/1  "<pC3>"
  Bus Creator2/1 -> LM_LR_Line06/1
  Signal Copy3/1 -> Bus Creator2/3  "pC2"
  Signal Copy6/1 -> Bus Creator2/5  "dDisStart"
  Signal Copy24/1 -> Bus Creator2/1  "pC0"
  Bus Selector2/1 -> Signal Copy24/1  "<pC0>"
  LM_Line06/1 -> Bus Selector2/1
  Bus Selector2/3 -> Signal Copy3/1  "<pC2>"
  Signal Copy4/1 -> Bus Creator2/6  "dDisEnd"
  Bus Selector2/5 -> Signal Copy6/1  "<dDisStart>"
  Bus Selector2/6 -> Signal Copy4/1  "<dDisEnd>"
  Bus Selector2/7 -> Signal Copy7/1  "<dQuality>"
  Bus Selector2/2 -> Signal Copy1/1  "<pC1>"
  Bus Selector2/8 -> Signal Copy5/1  "<fCamValid>"
  Signal Copy7/1 -> Bus Creator2/7  "dQuality"
  Signal Copy5/1 -> Bus Creator2/8  "fCamValid"
  Signal Copy2/1 -> Bus Creator2/4  "pC3"

== system PubIfDecisionTOS_MDL/TOS_20201112/TOS_2012080320/PP1128/ISV_InputSignalVerification/LM_SignalVerif/LM_LR_Bus/LM_LR_Line07 ==
  LM_Line07 : Inport
  Bus Creator2 : BusCreator  Inputs=8  OutDataTypeStr=Bus: TOS_LM_Line_bus  NonVirtualBus=on
      settings: InheritFromInputs=off
  Bus Selector2 : BusSelector  OutputSignals=pC0,pC1,pC2,pC3,dDisStart,dDisEnd,dQuality,fCamValid
  Signal Copy{1..7,24} (8 alike) : SignalConversion  OverrideOpt=off
  LM_LR_Line07 : Outport
  wires:
  Signal Copy2/1 -> Bus Creator2/4  "pC3"
  Signal Copy5/1 -> Bus Creator2/8  "fCamValid"
  Signal Copy7/1 -> Bus Creator2/7  "dQuality"
  Bus Selector2/8 -> Signal Copy5/1  "<fCamValid>"
  Bus Selector2/2 -> Signal Copy1/1  "<pC1>"
  Bus Selector2/7 -> Signal Copy7/1  "<dQuality>"
  Bus Selector2/6 -> Signal Copy4/1  "<dDisEnd>"
  Bus Selector2/5 -> Signal Copy6/1  "<dDisStart>"
  Signal Copy4/1 -> Bus Creator2/6  "dDisEnd"
  Bus Selector2/3 -> Signal Copy3/1  "<pC2>"
  LM_Line07/1 -> Bus Selector2/1
  Bus Selector2/1 -> Signal Copy24/1  "<pC0>"
  Signal Copy24/1 -> Bus Creator2/1  "pC0"
  Signal Copy6/1 -> Bus Creator2/5  "dDisStart"
  Signal Copy3/1 -> Bus Creator2/3  "pC2"
  Bus Creator2/1 -> LM_LR_Line07/1
  Bus Selector2/4 -> Signal Copy2/1  "<pC3>"
  Signal Copy1/1 -> Bus Creator2/2  "pC1"

== system PubIfDecisionTOS_MDL/TOS_20201112/TOS_2012080320/PP1128/ISV_InputSignalVerification/LM_SignalVerif/LM_LR_Bus/LM_LR_Line08 ==
  LM_Line08 : Inport
  Bus Creator2 : BusCreator  Inputs=8  OutDataTypeStr=Bus: TOS_LM_Line_bus  NonVirtualBus=on
      settings: InheritFromInputs=off
  Bus Selector2 : BusSelector  OutputSignals=pC0,pC1,pC2,pC3,dDisStart,dDisEnd,dQuality,fCamValid
  Signal Copy{1..7,24} (8 alike) : SignalConversion  OverrideOpt=off
  LM_LR_Line08 : Outport
  wires:
  Signal Copy1/1 -> Bus Creator2/2  "pC1"
  Bus Selector2/4 -> Signal Copy2/1  "<pC3>"
  Bus Creator2/1 -> LM_LR_Line08/1
  Signal Copy3/1 -> Bus Creator2/3  "pC2"
  Signal Copy6/1 -> Bus Creator2/5  "dDisStart"
  Signal Copy24/1 -> Bus Creator2/1  "pC0"
  Bus Selector2/1 -> Signal Copy24/1  "<pC0>"
  LM_Line08/1 -> Bus Selector2/1
  Bus Selector2/3 -> Signal Copy3/1  "<pC2>"
  Signal Copy4/1 -> Bus Creator2/6  "dDisEnd"
  Bus Selector2/5 -> Signal Copy6/1  "<dDisStart>"
  Bus Selector2/6 -> Signal Copy4/1  "<dDisEnd>"
  Bus Selector2/7 -> Signal Copy7/1  "<dQuality>"
  Bus Selector2/2 -> Signal Copy1/1  "<pC1>"
  Bus Selector2/8 -> Signal Copy5/1  "<fCamValid>"
  Signal Copy7/1 -> Bus Creator2/7  "dQuality"
  Signal Copy5/1 -> Bus Creator2/8  "fCamValid"
  Signal Copy2/1 -> Bus Creator2/4  "pC3"

== system PubIfDecisionTOS_MDL/TOS_20201112/TOS_2012080320/PP1128/ISV_InputSignalVerification/LM_SignalVerif/LM_RL_Bus/LM_RL_Line01 ==
  LM_Line01 : Inport
  Bus Creator2 : BusCreator  Inputs=8  OutDataTypeStr=Bus: TOS_LM_Line_bus  NonVirtualBus=on
      settings: InheritFromInputs=off
  Bus Selector2 : BusSelector  OutputSignals=pC0,pC1,pC2,pC3,dDisStart,dDisEnd,dQuality,fCamValid
  Signal Copy{1..7,24} (8 alike) : SignalConversion  OverrideOpt=off
  LM_RL_Line01 : Outport
  wires:
  Signal Copy1/1 -> Bus Creator2/2  "pC1"
  Bus Selector2/4 -> Signal Copy2/1  "<pC3>"
  Bus Creator2/1 -> LM_RL_Line01/1
  Signal Copy3/1 -> Bus Creator2/3  "pC2"
  Signal Copy6/1 -> Bus Creator2/5  "dDisStart"
  Signal Copy24/1 -> Bus Creator2/1  "pC0"
  Bus Selector2/1 -> Signal Copy24/1  "<pC0>"
  LM_Line01/1 -> Bus Selector2/1
  Bus Selector2/3 -> Signal Copy3/1  "<pC2>"
  Signal Copy4/1 -> Bus Creator2/6  "dDisEnd"
  Bus Selector2/5 -> Signal Copy6/1  "<dDisStart>"
  Bus Selector2/6 -> Signal Copy4/1  "<dDisEnd>"
  Bus Selector2/7 -> Signal Copy7/1  "<dQuality>"
  Bus Selector2/2 -> Signal Copy1/1  "<pC1>"
  Bus Selector2/8 -> Signal Copy5/1  "<fCamValid>"
  Signal Copy7/1 -> Bus Creator2/7  "dQuality"
  Signal Copy5/1 -> Bus Creator2/8  "fCamValid"
  Signal Copy2/1 -> Bus Creator2/4  "pC3"

== system PubIfDecisionTOS_MDL/TOS_20201112/TOS_2012080320/PP1128/ISV_InputSignalVerification/LM_SignalVerif/LM_RL_Bus/LM_RL_Line02 ==
  LM_Line02 : Inport
  Bus Creator2 : BusCreator  Inputs=8  OutDataTypeStr=Bus: TOS_LM_Line_bus  NonVirtualBus=on
      settings: InheritFromInputs=off
  Bus Selector2 : BusSelector  OutputSignals=pC0,pC1,pC2,pC3,dDisStart,dDisEnd,dQuality,fCamValid
  Signal Copy{1..7,24} (8 alike) : SignalConversion  OverrideOpt=off
  LM_RL_Line02 : Outport
  wires:
  Signal Copy2/1 -> Bus Creator2/4  "pC3"
  Signal Copy5/1 -> Bus Creator2/8  "fCamValid"
  Signal Copy7/1 -> Bus Creator2/7  "dQuality"
  Bus Selector2/8 -> Signal Copy5/1  "<fCamValid>"
  Bus Selector2/2 -> Signal Copy1/1  "<pC1>"
  Bus Selector2/7 -> Signal Copy7/1  "<dQuality>"
  Bus Selector2/6 -> Signal Copy4/1  "<dDisEnd>"
  Bus Selector2/5 -> Signal Copy6/1  "<dDisStart>"
  Signal Copy4/1 -> Bus Creator2/6  "dDisEnd"
  Bus Selector2/3 -> Signal Copy3/1  "<pC2>"
  LM_Line02/1 -> Bus Selector2/1
  Bus Selector2/1 -> Signal Copy24/1  "<pC0>"
  Signal Copy24/1 -> Bus Creator2/1  "pC0"
  Signal Copy6/1 -> Bus Creator2/5  "dDisStart"
  Signal Copy3/1 -> Bus Creator2/3  "pC2"
  Bus Creator2/1 -> LM_RL_Line02/1
  Bus Selector2/4 -> Signal Copy2/1  "<pC3>"
  Signal Copy1/1 -> Bus Creator2/2  "pC1"

== system PubIfDecisionTOS_MDL/TOS_20201112/TOS_2012080320/PP1128/ISV_InputSignalVerification/LM_SignalVerif/LM_RL_Bus/LM_RL_Line03 ==
  LM_Line03 : Inport
  Bus Creator2 : BusCreator  Inputs=8  OutDataTypeStr=Bus: TOS_LM_Line_bus  NonVirtualBus=on
      settings: InheritFromInputs=off
  Bus Selector2 : BusSelector  OutputSignals=pC0,pC1,pC2,pC3,dDisStart,dDisEnd,dQuality,fCamValid
  Signal Copy{1..7,24} (8 alike) : SignalConversion  OverrideOpt=off
  LM_RL_Line03 : Outport
  wires:
  Signal Copy1/1 -> Bus Creator2/2  "pC1"
  Bus Selector2/4 -> Signal Copy2/1  "<pC3>"
  Bus Creator2/1 -> LM_RL_Line03/1
  Signal Copy3/1 -> Bus Creator2/3  "pC2"
  Signal Copy6/1 -> Bus Creator2/5  "dDisStart"
  Signal Copy24/1 -> Bus Creator2/1  "pC0"
  Bus Selector2/1 -> Signal Copy24/1  "<pC0>"
  LM_Line03/1 -> Bus Selector2/1
  Bus Selector2/3 -> Signal Copy3/1  "<pC2>"
  Signal Copy4/1 -> Bus Creator2/6  "dDisEnd"
  Bus Selector2/5 -> Signal Copy6/1  "<dDisStart>"
  Bus Selector2/6 -> Signal Copy4/1  "<dDisEnd>"
  Bus Selector2/7 -> Signal Copy7/1  "<dQuality>"
  Bus Selector2/2 -> Signal Copy1/1  "<pC1>"
  Bus Selector2/8 -> Signal Copy5/1  "<fCamValid>"
  Signal Copy7/1 -> Bus Creator2/7  "dQuality"
  Signal Copy5/1 -> Bus Creator2/8  "fCamValid"
  Signal Copy2/1 -> Bus Creator2/4  "pC3"

== system PubIfDecisionTOS_MDL/TOS_20201112/TOS_2012080320/PP1128/ISV_InputSignalVerification/LM_SignalVerif/LM_RL_Bus/LM_RL_Line04 ==
  LM_Line04 : Inport
  Bus Creator2 : BusCreator  Inputs=8  OutDataTypeStr=Bus: TOS_LM_Line_bus  NonVirtualBus=on
      settings: InheritFromInputs=off
  Bus Selector2 : BusSelector  OutputSignals=pC0,pC1,pC2,pC3,dDisStart,dDisEnd,dQuality,fCamValid
  Signal Copy{1..7,24} (8 alike) : SignalConversion  OverrideOpt=off
  LM_RL_Line04 : Outport
  wires:
  Signal Copy2/1 -> Bus Creator2/4  "pC3"
  Signal Copy5/1 -> Bus Creator2/8  "fCamValid"
  Signal Copy7/1 -> Bus Creator2/7  "dQuality"
  Bus Selector2/8 -> Signal Copy5/1  "<fCamValid>"
  Bus Selector2/2 -> Signal Copy1/1  "<pC1>"
  Bus Selector2/7 -> Signal Copy7/1  "<dQuality>"
  Bus Selector2/6 -> Signal Copy4/1  "<dDisEnd>"
  Bus Selector2/5 -> Signal Copy6/1  "<dDisStart>"
  Signal Copy4/1 -> Bus Creator2/6  "dDisEnd"
  Bus Selector2/3 -> Signal Copy3/1  "<pC2>"
  LM_Line04/1 -> Bus Selector2/1
  Bus Selector2/1 -> Signal Copy24/1  "<pC0>"
  Signal Copy24/1 -> Bus Creator2/1  "pC0"
  Signal Copy6/1 -> Bus Creator2/5  "dDisStart"
  Signal Copy3/1 -> Bus Creator2/3  "pC2"
  Bus Creator2/1 -> LM_RL_Line04/1
  Bus Selector2/4 -> Signal Copy2/1  "<pC3>"
  Signal Copy1/1 -> Bus Creator2/2  "pC1"
